simulink model "punto6b1"  (Simulink 5.0)
settings: Solver=ode45  StartTime=0.0  StopTime=10  RelTol=1e-3
libraries: dspsrcs4 x1
settings Model: LastModifiedBy=Juan

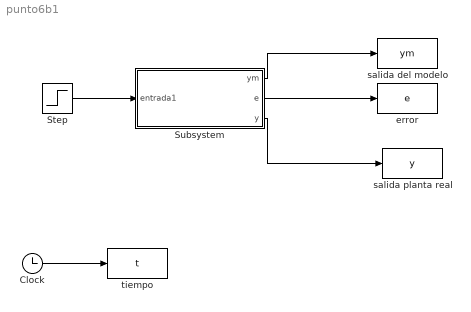
== system punto6b1 ==
  Clock : Clock
      settings: Decimation=10
  Step : Step  Time=0  After=10  SampleTime=0
  Subsystem : Subsystem  mask{kp=1, km=1, g=0.1, var=0, titainicial1=1.14, titainicial2=-0.65}
      mask prompts: kp "ganancia de la planta real (kp)"; km "ganancia del modelo (km)"; g "gama"; var "varianza del ruido gaussiano"; titainicial1 "valor inicial de tita 1"; titainicial2 "valor inicial de tita 2"
      mask Display: disp('Sistema')
  error : ToWorkspace  VariableName=e  SampleTime=-1  SaveFormat=Array
  salida del modelo : ToWorkspace  VariableName=ym  SampleTime=-1  SaveFormat=Array
  salida planta real : ToWorkspace  VariableName=y  SampleTime=-1  SaveFormat=Array
  tiempo : ToWorkspace  VariableName=t  SampleTime=-1  SaveFormat=Array
  wires:
  Clock/1 -> tiempo/1
  Subsystem/1(ym) -> salida del modelo/1
  Subsystem/2(e) -> error/1
  Subsystem/3(y) -> salida planta real/1
  Step/1 -> Subsystem/1(entrada1)

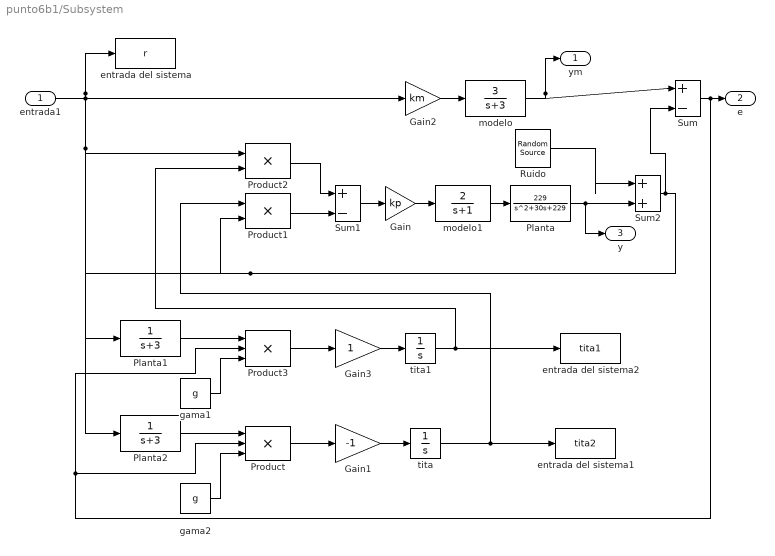
== system punto6b1/Subsystem ==
  entrada1 : Inport
  Gain : Gain  Gain=kp  SaturateOnIntegerOverflow=on
  Gain1 : Gain  Gain=-1  SaturateOnIntegerOverflow=on
  Gain2 : Gain  Gain=km  SaturateOnIntegerOverflow=on
  Gain3 : Gain  SaturateOnIntegerOverflow=on
  Planta : TransferFcn  Numerator=229  Denominator=[1 30 229]
  Planta1 : TransferFcn  Numerator=1  Denominator=[1 3]
  Planta2 : TransferFcn  Numerator=1  Denominator=[1 3]
  Product : Product  Inputs=3  SaturateOnIntegerOverflow=on
  Product1 : Product  SaturateOnIntegerOverflow=on
  Product2 : Product  SaturateOnIntegerOverflow=on
  Product3 : Product  Inputs=3  SaturateOnIntegerOverflow=on
  Ruido : dspsrcs4/Random Source  SrcType=Gaussian  NormMethod=Ziggurat  CltLength=12  Min=0  Max=1  Mean=0  Var=var  RepMode=Not repeatable  Seed=1  Inherit=off  SampMode=Continuous  SampTime=1  SampFrame=1  DataType=Double  OutComplex=Real
  Sum : Sum  Inputs=|+-  SaturateOnIntegerOverflow=on
  Sum1 : Sum  Inputs=|+-  SaturateOnIntegerOverflow=on
  Sum2 : Sum  Inputs=|++  SaturateOnIntegerOverflow=on
  entrada del sistema : ToWorkspace  VariableName=r  SampleTime=-1  SaveFormat=Array
  entrada del sistema1 : ToWorkspace  VariableName=tita2  SampleTime=-1  SaveFormat=Array
  entrada del sistema2 : ToWorkspace  VariableName=tita1  SampleTime=-1  SaveFormat=Array
  gama1 : Constant  Value=g
  gama2 : Constant  Value=g
  modelo : TransferFcn  Numerator=3  Denominator=[1 3]
  modelo1 : TransferFcn  Numerator=2  Denominator=[1 1]
  tita : Integrator  InitialCondition=titainicial2
  tita1 : Integrator  InitialCondition=titainicial1
  ym : Outport
  e : Outport  Port=2
  y : Outport  Port=3
  wires:
  modelo/1 -> ym/1, Sum/1
  Planta/1 -> y/1, Sum2/2
  Gain1/1 -> tita/1
  Sum/1 -> e/1, Product3/2, Product/2
  Gain2/1 -> modelo/1
  Gain/1 -> modelo1/1
  entrada1/1 -> Gain2/1, entrada del sistema/1, Product2/1, Planta1/1
  Sum1/1 -> Gain/1
  Product1/1 -> Sum1/2
  Product2/1 -> Sum1/1
  Ruido/1 -> Sum2/1
  Sum2/1 -> Sum/2, Product1/2, Planta2/1
  Planta1/1 -> Product3/1
  gama1/1 -> Product3/3
  Product3/1 -> Gain3/1
  Gain3/1 -> tita1/1
  tita1/1 -> Product2/2, entrada del sistema2/1
  Product/1 -> Gain1/1
  tita/1 -> Product1/1, entrada del sistema1/1
  Planta2/1 -> Product/1
  gama2/1 -> Product/3
  modelo1/1 -> Planta/1
